simulink model "Md58StEnCtrl"  (R2018b)
settings: Solver=FixedStepDiscrete  StartTime=0.0  StopTime=10.0  FixedStep=0.01  RelTol=1e-3
undefined symbols (not defined in the file or in its folder): data, KeSMSuFirstRwStBackPosDelta_Val, KeSMSuFirstRwStCushFoldPosDelta_Val, KeSMSuFirstRwStFwdBkwdPosDelta_Val, KeSMSw4SSecRwLtStLgrstOtwdInwdClosePos1_Val, KeSMSw4SSecRwLtStLgrstUpwdDnwdClosePos1_Val, KeSMSw4SSecRwLtStLgrstUpwdDnwdClosePos2_Val, KeSMSw4SSecRwLtStLgrstUpwdDnwdOpenPos1_Val, PassStBkReclnEn_Clear, PassStBkReclnEn_Set, PassStCshnFldEn_Clear, PassStCshnFldEn_Set, PassStFwdBkwdEn_Clear, PassStFwdBkwdEn_Set, SecRwRtStBkReclnEn_Clear, SecRwRtStBkReclnEn_Set, SecRwRtStFwdBkwdEn_Clear, SecRwRtStFwdBkwdEn_Set, SecRwRtStLgrstInwdOtwdEn_Clear, SecRwRtStLgrstInwdOtwdEn_Set, SecRwRtStLgrstUpwdDnwdEn_Clear, SecRwRtStLgrstUpwdDnwdEn_Set, ThdRwLtStBkReclnEn_Clear, ThdRwLtStBkReclnEn_Set, ThdRwLtStFwdBkwdEn_Clear, ThdRwLtStFwdBkwdEn_Set, ThdRwRtStBkReclnEn_Clear, ThdRwRtStBkReclnEn_Set, ThdRwRtStFwdBkwdEn_Clear, ThdRwRtStFwdBkwdEn_Set, ZeroREn_Clear, ZeroREn_Set
libraries: simulink x1
(part 1 of 2)
settings Model: Creator=sn2xws  LastModifiedBy=sn2xws
settings Model: ModifiedHistory=|
  | 2024.10.21 V3.0.0 新增Md58
  | 2024.11.18 V3.0.1 CR946473
  | 2024.112.4  V3.0.2 单元测试发现的副驾到位置判断问题
settings DataIOCC: SaveFormat=StructureWithTime
settings OptimizationCC: DefaultParameterBehavior=Inlined  EnhancedBackFolding=on  PassReuseOutputArgsAs=Individual arguments  ZeroExternalMemoryAtStartup=off  ZeroInternalMemoryAtStartup=off  OptimizeBlockOrder=speed  DifferentSizesBufferReuse=on  OptimizationCustomize=off
settings DebuggingCC: ParameterTunabilityLossMsg=error
settings SFSimCC: MATLABDynamicMemAlloc=off
settings RTWCC: SystemTargetFile=autosar.tlc  GenCodeOnly=on  TemplateMakefile=ert_default_tmf  Description=AUTOSAR  GenerateReport=on  IncludeHyperlinkInReport=on  LaunchReport=on  GenerateTraceInfo=on  GenerateTraceReport=on  GenerateTraceReportSl=on  GenerateTraceReportSf=on  GenerateTraceReportEml=on
settings CodeAppCC: ForceParamTrailComments=on  IgnoreCustomStorageClasses=off  OperatorAnnotations=on  SimulinkDataObjDesc=on  SFDataObjDesc=on  InsertBlockDesc=on
settings STFCustomTargetCC: TargetLangStandard=C99 (ISO)  MultiwordLength=256  ParMdlRefBuildCompliant=on  CompOptLevelCompliant=on  IncludeMdlTerminateFcn=off  CombineOutputUpdateFcns=on  SuppressErrorStatus=on  ERTCustomFileBanners=on  SupportNonFinite=off  SupportComplex=off  SupportContinuousTime=off  SupportNonInlinedSFcns=off  RemoveResetFunc=on  MATLABClassNameForMDSCustomization=Simulink.SoftwareTarget.ERTCustomization  AutosarCompliant=on  UseToolchainInfoCompliant=on  LookupTableObjectStructAxisOrder=2,1,3,4,...  LUTObjectStructOrderEvenSpacing=Size,Table,Breakpoints  SystemTargetFile=autosar.tlc
settings ERTTargetCC: TargetLangStandard=C99 (ISO)  ConcurrentExecutionCompliant=off  IncludeMdlTerminateFcn=off  SuppressErrorStatus=on  SupportNonFinite=off  SupportComplex=off  ModelStepFunctionPrototypeControlCompliant=off  CPPClassGenCompliant=off  AutosarCompliant=on  LookupTableObjectStructAxisOrder=2,1,3,4,...  LUTObjectStructOrderEvenSpacing=Size,Table,Breakpoints  InlinedParameterPlacement=NonHierarchical  ERTCustomFileTemplate=example_file_process.tlc  ERTFilePackagingFormat=Compact

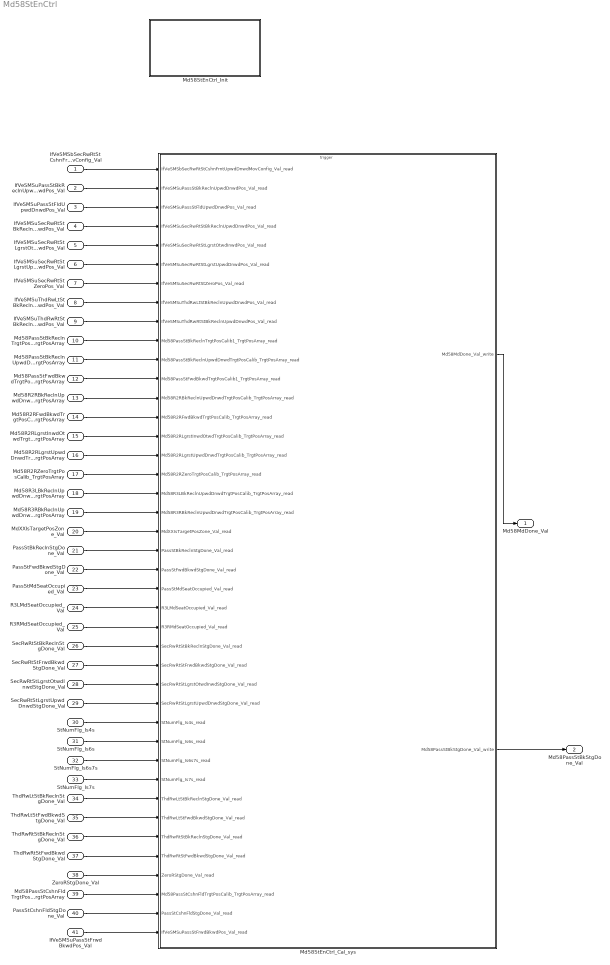
== system Md58StEnCtrl ==
  IfVeSMSbSecRwRtStCshnFrntUpwdDnwdMovConfig_Val : Inport  OutDataTypeStr=boolean  PortDimensions=1
  IfVeSMSuPassStBkReclnUpwdDnwdPos_Val : Inport  Port=2  OutDataTypeStr=uint16  PortDimensions=1
  IfVeSMSuPassStFldUpwdDnwdPos_Val : Inport  Port=3  OutDataTypeStr=uint16  PortDimensions=1
  IfVeSMSuSecRwRtStBkReclnUpwdDnwdPos_Val : Inport  Port=4  OutDataTypeStr=uint16  PortDimensions=1
  IfVeSMSuSecRwRtStLgrstOtwdInwdPos_Val : Inport  Port=5  OutDataTypeStr=uint16  PortDimensions=1
  IfVeSMSuSecRwRtStLgrstUpwdDnwdPos_Val : Inport  Port=6  OutDataTypeStr=uint16  PortDimensions=1
  IfVeSMSuSecRwRtStZeroPos_Val : Inport  Port=7  OutDataTypeStr=uint16  PortDimensions=1
  IfVeSMSuThdRwLtStBkReclnUpwdDnwdPos_Val : Inport  Port=8  OutDataTypeStr=uint16  PortDimensions=1
  IfVeSMSuThdRwRtStBkReclnUpwdDnwdPos_Val : Inport  Port=9  OutDataTypeStr=uint16  PortDimensions=1
  Md58PassStBkReclnTrgtPosCalib1_TrgtPosArray : Inport  Description=|  Port=10  OutDataTypeStr=uint16  PortDimensions=3
      | 0:Pos
      | 1:Max
      | 2:Min
  Md58PassStBkReclnUpwdDnwdTrgtPosCalib_TrgtPosArray : Inport  Description=|  Port=11  OutDataTypeStr=uint16  PortDimensions=3
      | 0:Pos
      | 1:Max
      | 2:Min
  Md58PassStFwdBkwdTrgtPosCalib1_TrgtPosArray : Inport  Description=|  Port=12  OutDataTypeStr=uint16  PortDimensions=3
      | 0:Pos
      | 1:Max
      | 2:Min
  Md58R2RBkReclnUpwdDnwdTrgtPosCalib_TrgtPosArray : Inport  Description=|  Port=13  OutDataTypeStr=uint16  PortDimensions=3
      | 0:Pos
      | 1:Max
      | 2:Min
  Md58R2RFwdBkwdTrgtPosCalib_TrgtPosArray : Inport  Description=|  Port=14  OutDataTypeStr=uint16  PortDimensions=3
      | 0:Pos
      | 1:Max
      | 2:Min
  Md58R2RLgrstInwdOtwdTrgtPosCalib_TrgtPosArray : Inport  Description=|  Port=15  OutDataTypeStr=uint16  PortDimensions=3
      | 0:Pos
      | 1:Max
      | 2:Min
  Md58R2RLgrstUpwdDnwdTrgtPosCalib_TrgtPosArray : Inport  Description=|  Port=16  OutDataTypeStr=uint16  PortDimensions=3
      | 0:Pos
      | 1:Max
      | 2:Min
  Md58R2RZeroTrgtPosCalib_TrgtPosArray : Inport  Description=|  Port=17  OutDataTypeStr=uint16  PortDimensions=3
      | 0:Pos
      | 1:Max
      | 2:Min
  Md58R3LBkReclnUpwdDnwdTrgtPosCalib_TrgtPosArray : Inport  Description=|  Port=18  OutDataTypeStr=uint16  PortDimensions=3
      | 0:Pos
      | 1:Max
      | 2:Min
  Md58R3RBkReclnUpwdDnwdTrgtPosCalib_TrgtPosArray : Inport  Description=|  Port=19  OutDataTypeStr=uint16  PortDimensions=3
      | 0:Pos
      | 1:Max
      | 2:Min
  MdXXIsTargetPosZone_Val : Inport  Port=20  OutDataTypeStr=uint32  PortDimensions=1
  PassStBkReclnStgDone_Val : Inport  Port=21  OutDataTypeStr=boolean  PortDimensions=1
  PassStFwdBkwdStgDone_Val : Inport  Port=22  OutDataTypeStr=boolean  PortDimensions=1
  PassStMdSeatOccupied_Val : Inport  Port=23  OutDataTypeStr=boolean  PortDimensions=1
  R3LMdSeatOccupied_Val : Inport  Port=24  OutDataTypeStr=boolean  PortDimensions=1
  R3RMdSeatOccupied_Val : Inport  Port=25  OutDataTypeStr=boolean  PortDimensions=1
  SecRwRtStBkReclnStgDone_Val : Inport  Port=26  OutDataTypeStr=boolean  PortDimensions=1
  SecRwRtStFrwdBkwdStgDone_Val : Inport  Port=27  OutDataTypeStr=boolean  PortDimensions=1
  SecRwRtStLgrstOtwdInwdStgDone_Val : Inport  Port=28  OutDataTypeStr=boolean  PortDimensions=1
  SecRwRtStLgrstUpwdDnwdStgDone_Val : Inport  Port=29  OutDataTypeStr=boolean  PortDimensions=1
  StNumFlg_Is4s : Inport  Port=30  OutDataTypeStr=boolean  PortDimensions=1
  StNumFlg_Is6s : Inport  Port=31  OutDataTypeStr=boolean  PortDimensions=1
  StNumFlg_Is6s7s : Inport  Port=32  OutDataTypeStr=boolean  PortDimensions=1
  StNumFlg_Is7s : Inport  Port=33  OutDataTypeStr=boolean  PortDimensions=1
  ThdRwLtStBkReclnStgDone_Val : Inport  Port=34  OutDataTypeStr=boolean  PortDimensions=1
  ThdRwLtStFwdBkwdStgDone_Val : Inport  Port=35  OutDataTypeStr=boolean  PortDimensions=1
  ThdRwRtStBkReclnStgDone_Val : Inport  Port=36  OutDataTypeStr=boolean  PortDimensions=1
  ThdRwRtStFwdBkwdStgDone_Val : Inport  Port=37  OutDataTypeStr=boolean  PortDimensions=1
  ZeroRStgDone_Val : Inport  Port=38  OutDataTypeStr=boolean  PortDimensions=1
  Md58PassStCshnFldTrgtPosCalib_TrgtPosArray : Inport  Description=|  Port=39  OutDataTypeStr=uint16  PortDimensions=3
      | 0:Pos
      | 1:Max
      | 2:Min
  PassStCshnFldStgDone_Val : Inport  Port=40  OutDataTypeStr=boolean  PortDimensions=1
  IfVeSMSuPassStFrwdBkwdPos_Val : Inport  Port=41  OutDataTypeStr=uint16  PortDimensions=1
  Md58StEnCtrl_Cal_sys : Subsystem
  Md58StEnCtrl_Init : Subsystem
  Md58MdDone_Val : Outport  OutDataTypeStr=uint8  PortDimensions=1
  Md58PassStBkStgDone_Val : Outport  Port=2  OutDataTypeStr=boolean  PortDimensions=1
  wires:
  IfVeSMSbSecRwRtStCshnFrntUpwdDnwdMovConfig_Val/1 -> Md58StEnCtrl_Cal_sys/1(IfVeSMSbSecRwRtStCshnFrntUpwdDnwdMovConfig_Val_read)
  IfVeSMSuPassStBkReclnUpwdDnwdPos_Val/1 -> Md58StEnCtrl_Cal_sys/2(IfVeSMSuPassStBkReclnUpwdDnwdPos_Val_read)
  IfVeSMSuPassStFldUpwdDnwdPos_Val/1 -> Md58StEnCtrl_Cal_sys/3(IfVeSMSuPassStFldUpwdDnwdPos_Val_read)
  IfVeSMSuSecRwRtStBkReclnUpwdDnwdPos_Val/1 -> Md58StEnCtrl_Cal_sys/4(IfVeSMSuSecRwRtStBkReclnUpwdDnwdPos_Val_read)
  IfVeSMSuSecRwRtStLgrstOtwdInwdPos_Val/1 -> Md58StEnCtrl_Cal_sys/5(IfVeSMSuSecRwRtStLgrstOtwdInwdPos_Val_read)
  IfVeSMSuSecRwRtStLgrstUpwdDnwdPos_Val/1 -> Md58StEnCtrl_Cal_sys/6(IfVeSMSuSecRwRtStLgrstUpwdDnwdPos_Val_read)
  IfVeSMSuSecRwRtStZeroPos_Val/1 -> Md58StEnCtrl_Cal_sys/7(IfVeSMSuSecRwRtStZeroPos_Val_read)
  IfVeSMSuThdRwLtStBkReclnUpwdDnwdPos_Val/1 -> Md58StEnCtrl_Cal_sys/8(IfVeSMSuThdRwLtStBkReclnUpwdDnwdPos_Val_read)
  IfVeSMSuThdRwRtStBkReclnUpwdDnwdPos_Val/1 -> Md58StEnCtrl_Cal_sys/9(IfVeSMSuThdRwRtStBkReclnUpwdDnwdPos_Val_read)
  Md58PassStBkReclnTrgtPosCalib1_TrgtPosArray/1 -> Md58StEnCtrl_Cal_sys/10(Md58PassStBkReclnTrgtPosCalib1_TrgtPosArray_read)
  Md58PassStBkReclnUpwdDnwdTrgtPosCalib_TrgtPosArray/1 -> Md58StEnCtrl_Cal_sys/11(Md58PassStBkReclnUpwdDnwdTrgtPosCalib_TrgtPosArray_read)
  Md58PassStFwdBkwdTrgtPosCalib1_TrgtPosArray/1 -> Md58StEnCtrl_Cal_sys/12(Md58PassStFwdBkwdTrgtPosCalib1_TrgtPosArray_read)
  Md58R2RBkReclnUpwdDnwdTrgtPosCalib_TrgtPosArray/1 -> Md58StEnCtrl_Cal_sys/13(Md58R2RBkReclnUpwdDnwdTrgtPosCalib_TrgtPosArray_read)
  Md58R2RFwdBkwdTrgtPosCalib_TrgtPosArray/1 -> Md58StEnCtrl_Cal_sys/14(Md58R2RFwdBkwdTrgtPosCalib_TrgtPosArray_read)
  Md58R2RLgrstInwdOtwdTrgtPosCalib_TrgtPosArray/1 -> Md58StEnCtrl_Cal_sys/15(Md58R2RLgrstInwdOtwdTrgtPosCalib_TrgtPosArray_read)
  Md58R2RLgrstUpwdDnwdTrgtPosCalib_TrgtPosArray/1 -> Md58StEnCtrl_Cal_sys/16(Md58R2RLgrstUpwdDnwdTrgtPosCalib_TrgtPosArray_read)
  Md58R2RZeroTrgtPosCalib_TrgtPosArray/1 -> Md58StEnCtrl_Cal_sys/17(Md58R2RZeroTrgtPosCalib_TrgtPosArray_read)
  Md58R3LBkReclnUpwdDnwdTrgtPosCalib_TrgtPosArray/1 -> Md58StEnCtrl_Cal_sys/18(Md58R3LBkReclnUpwdDnwdTrgtPosCalib_TrgtPosArray_read)
  Md58R3RBkReclnUpwdDnwdTrgtPosCalib_TrgtPosArray/1 -> Md58StEnCtrl_Cal_sys/19(Md58R3RBkReclnUpwdDnwdTrgtPosCalib_TrgtPosArray_read)
  MdXXIsTargetPosZone_Val/1 -> Md58StEnCtrl_Cal_sys/20(MdXXIsTargetPosZone_Val_read)
  PassStBkReclnStgDone_Val/1 -> Md58StEnCtrl_Cal_sys/21(PassStBkReclnStgDone_Val_read)
  PassStFwdBkwdStgDone_Val/1 -> Md58StEnCtrl_Cal_sys/22(PassStFwdBkwdStgDone_Val_read)
  PassStMdSeatOccupied_Val/1 -> Md58StEnCtrl_Cal_sys/23(PassStMdSeatOccupied_Val_read)
  R3LMdSeatOccupied_Val/1 -> Md58StEnCtrl_Cal_sys/24(R3LMdSeatOccupied_Val_read)
  R3RMdSeatOccupied_Val/1 -> Md58StEnCtrl_Cal_sys/25(R3RMdSeatOccupied_Val_read)
  SecRwRtStBkReclnStgDone_Val/1 -> Md58StEnCtrl_Cal_sys/26(SecRwRtStBkReclnStgDone_Val_read)
  SecRwRtStFrwdBkwdStgDone_Val/1 -> Md58StEnCtrl_Cal_sys/27(SecRwRtStFrwdBkwdStgDone_Val_read)
  SecRwRtStLgrstOtwdInwdStgDone_Val/1 -> Md58StEnCtrl_Cal_sys/28(SecRwRtStLgrstOtwdInwdStgDone_Val_read)
  SecRwRtStLgrstUpwdDnwdStgDone_Val/1 -> Md58StEnCtrl_Cal_sys/29(SecRwRtStLgrstUpwdDnwdStgDone_Val_read)
  StNumFlg_Is4s/1 -> Md58StEnCtrl_Cal_sys/30(StNumFlg_Is4s_read)
  StNumFlg_Is6s/1 -> Md58StEnCtrl_Cal_sys/31(StNumFlg_Is6s_read)
  StNumFlg_Is6s7s/1 -> Md58StEnCtrl_Cal_sys/32(StNumFlg_Is6s7s_read)
  StNumFlg_Is7s/1 -> Md58StEnCtrl_Cal_sys/33(StNumFlg_Is7s_read)
  ThdRwLtStBkReclnStgDone_Val/1 -> Md58StEnCtrl_Cal_sys/34(ThdRwLtStBkReclnStgDone_Val_read)
  ThdRwLtStFwdBkwdStgDone_Val/1 -> Md58StEnCtrl_Cal_sys/35(ThdRwLtStFwdBkwdStgDone_Val_read)
  ThdRwRtStBkReclnStgDone_Val/1 -> Md58StEnCtrl_Cal_sys/36(ThdRwRtStBkReclnStgDone_Val_read)
  ThdRwRtStFwdBkwdStgDone_Val/1 -> Md58StEnCtrl_Cal_sys/37(ThdRwRtStFwdBkwdStgDone_Val_read)
  ZeroRStgDone_Val/1 -> Md58StEnCtrl_Cal_sys/38(ZeroRStgDone_Val_read)
  Md58StEnCtrl_Cal_sys/1(Md58MdDone_Val_write) -> Md58MdDone_Val/1
  Md58PassStCshnFldTrgtPosCalib_TrgtPosArray/1 -> Md58StEnCtrl_Cal_sys/39(Md58PassStCshnFldTrgtPosCalib_TrgtPosArray_read)
  PassStCshnFldStgDone_Val/1 -> Md58StEnCtrl_Cal_sys/40(PassStCshnFldStgDone_Val_read)
  IfVeSMSuPassStFrwdBkwdPos_Val/1 -> Md58StEnCtrl_Cal_sys/41(IfVeSMSuPassStFrwdBkwdPos_Val_read)
  Md58StEnCtrl_Cal_sys/2(Md58PassStBkStgDone_Val_write) -> Md58PassStBkStgDone_Val/1

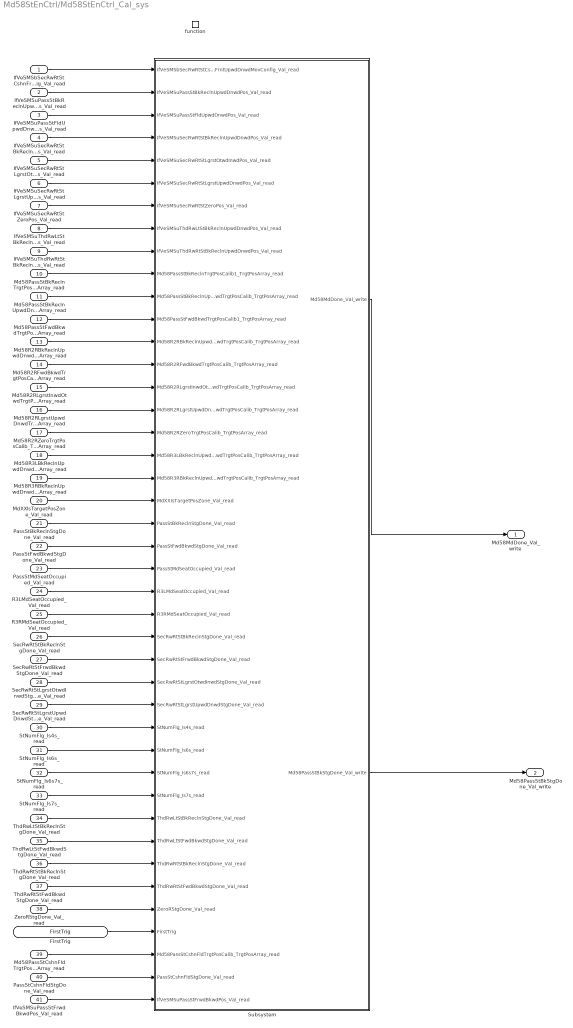
== system Md58StEnCtrl/Md58StEnCtrl_Cal_sys ==
  IfVeSMSbSecRwRtStCshnFrntUpwdDnwdMovConfig_Val_read : Inport
  IfVeSMSuPassStBkReclnUpwdDnwdPos_Val_read : Inport  Port=2
  IfVeSMSuPassStFldUpwdDnwdPos_Val_read : Inport  Port=3
  IfVeSMSuSecRwRtStBkReclnUpwdDnwdPos_Val_read : Inport  Port=4
  IfVeSMSuSecRwRtStLgrstOtwdInwdPos_Val_read : Inport  Port=5
  IfVeSMSuSecRwRtStLgrstUpwdDnwdPos_Val_read : Inport  Port=6
  IfVeSMSuSecRwRtStZeroPos_Val_read : Inport  Port=7
  IfVeSMSuThdRwLtStBkReclnUpwdDnwdPos_Val_read : Inport  Port=8
  IfVeSMSuThdRwRtStBkReclnUpwdDnwdPos_Val_read : Inport  Port=9
  Md58PassStBkReclnTrgtPosCalib1_TrgtPosArray_read : Inport  Port=10
  Md58PassStBkReclnUpwdDnwdTrgtPosCalib_TrgtPosArray_read : Inport  Port=11
  Md58PassStFwdBkwdTrgtPosCalib1_TrgtPosArray_read : Inport  Port=12
  Md58R2RBkReclnUpwdDnwdTrgtPosCalib_TrgtPosArray_read : Inport  Port=13
  Md58R2RFwdBkwdTrgtPosCalib_TrgtPosArray_read : Inport  Port=14
  Md58R2RLgrstInwdOtwdTrgtPosCalib_TrgtPosArray_read : Inport  Port=15
  Md58R2RLgrstUpwdDnwdTrgtPosCalib_TrgtPosArray_read : Inport  Port=16
  Md58R2RZeroTrgtPosCalib_TrgtPosArray_read : Inport  Port=17
  Md58R3LBkReclnUpwdDnwdTrgtPosCalib_TrgtPosArray_read : Inport  Port=18
  Md58R3RBkReclnUpwdDnwdTrgtPosCalib_TrgtPosArray_read : Inport  Port=19
  MdXXIsTargetPosZone_Val_read : Inport  Port=20
  PassStBkReclnStgDone_Val_read : Inport  Port=21
  PassStFwdBkwdStgDone_Val_read : Inport  Port=22
  PassStMdSeatOccupied_Val_read : Inport  Port=23
  R3LMdSeatOccupied_Val_read : Inport  Port=24
  R3RMdSeatOccupied_Val_read : Inport  Port=25
  SecRwRtStBkReclnStgDone_Val_read : Inport  Port=26
  SecRwRtStFrwdBkwdStgDone_Val_read : Inport  Port=27
  SecRwRtStLgrstOtwdInwdStgDone_Val_read : Inport  Port=28
  SecRwRtStLgrstUpwdDnwdStgDone_Val_read : Inport  Port=29
  StNumFlg_Is4s_read : Inport  Port=30
  StNumFlg_Is6s_read : Inport  Port=31
  StNumFlg_Is6s7s_read : Inport  Port=32
  StNumFlg_Is7s_read : Inport  Port=33
  ThdRwLtStBkReclnStgDone_Val_read : Inport  Port=34
  ThdRwLtStFwdBkwdStgDone_Val_read : Inport  Port=35
  ThdRwRtStBkReclnStgDone_Val_read : Inport  Port=36
  ThdRwRtStFwdBkwdStgDone_Val_read : Inport  Port=37
  ZeroRStgDone_Val_read : Inport  Port=38
  Md58PassStCshnFldTrgtPosCalib_TrgtPosArray_read : Inport  Port=39
  PassStCshnFldStgDone_Val_read : Inport  Port=40
  IfVeSMSuPassStFrwdBkwdPos_Val_read : Inport  Port=41
  function : TriggerPort  TriggerType=function-call  IsSimulinkFunction=on  FunctionName=Md58StEnCtrl_Cal  VariantControl=(inherit)
  Subsystem : Subsystem
  FirstTrig : ArgIn  OutDataTypeStr=boolean  ArgumentName=FirstTrig
  Md58MdDone_Val_write : Outport
      settings: EnsureOutportIsVirtual=on
  Md58PassStBkStgDone_Val_write : Outport  Port=2
      settings: EnsureOutportIsVirtual=on
  wires:
  IfVeSMSbSecRwRtStCshnFrntUpwdDnwdMovConfig_Val_read/1 -> Subsystem/1(IfVeSMSbSecRwRtStCshnFrntUpwdDnwdMovConfig_Val_read)
  IfVeSMSuPassStBkReclnUpwdDnwdPos_Val_read/1 -> Subsystem/2(IfVeSMSuPassStBkReclnUpwdDnwdPos_Val_read)
  IfVeSMSuPassStFldUpwdDnwdPos_Val_read/1 -> Subsystem/3(IfVeSMSuPassStFldUpwdDnwdPos_Val_read)
  IfVeSMSuSecRwRtStBkReclnUpwdDnwdPos_Val_read/1 -> Subsystem/4(IfVeSMSuSecRwRtStBkReclnUpwdDnwdPos_Val_read)
  IfVeSMSuSecRwRtStLgrstOtwdInwdPos_Val_read/1 -> Subsystem/5(IfVeSMSuSecRwRtStLgrstOtwdInwdPos_Val_read)
  IfVeSMSuSecRwRtStLgrstUpwdDnwdPos_Val_read/1 -> Subsystem/6(IfVeSMSuSecRwRtStLgrstUpwdDnwdPos_Val_read)
  IfVeSMSuSecRwRtStZeroPos_Val_read/1 -> Subsystem/7(IfVeSMSuSecRwRtStZeroPos_Val_read)
  IfVeSMSuThdRwLtStBkReclnUpwdDnwdPos_Val_read/1 -> Subsystem/8(IfVeSMSuThdRwLtStBkReclnUpwdDnwdPos_Val_read)
  IfVeSMSuThdRwRtStBkReclnUpwdDnwdPos_Val_read/1 -> Subsystem/9(IfVeSMSuThdRwRtStBkReclnUpwdDnwdPos_Val_read)
  Md58PassStBkReclnTrgtPosCalib1_TrgtPosArray_read/1 -> Subsystem/10(Md58PassStBkReclnTrgtPosCalib1_TrgtPosArray_read)
  Md58PassStBkReclnUpwdDnwdTrgtPosCalib_TrgtPosArray_read/1 -> Subsystem/11(Md58PassStBkReclnUpwdDnwdTrgtPosCalib_TrgtPosArray_read)
  Md58PassStFwdBkwdTrgtPosCalib1_TrgtPosArray_read/1 -> Subsystem/12(Md58PassStFwdBkwdTrgtPosCalib1_TrgtPosArray_read)
  Md58R2RBkReclnUpwdDnwdTrgtPosCalib_TrgtPosArray_read/1 -> Subsystem/13(Md58R2RBkReclnUpwdDnwdTrgtPosCalib_TrgtPosArray_read)
  Md58R2RFwdBkwdTrgtPosCalib_TrgtPosArray_read/1 -> Subsystem/14(Md58R2RFwdBkwdTrgtPosCalib_TrgtPosArray_read)
  Md58R2RLgrstInwdOtwdTrgtPosCalib_TrgtPosArray_read/1 -> Subsystem/15(Md58R2RLgrstInwdOtwdTrgtPosCalib_TrgtPosArray_read)
  Md58R2RLgrstUpwdDnwdTrgtPosCalib_TrgtPosArray_read/1 -> Subsystem/16(Md58R2RLgrstUpwdDnwdTrgtPosCalib_TrgtPosArray_read)
  Md58R2RZeroTrgtPosCalib_TrgtPosArray_read/1 -> Subsystem/17(Md58R2RZeroTrgtPosCalib_TrgtPosArray_read)
  Md58R3LBkReclnUpwdDnwdTrgtPosCalib_TrgtPosArray_read/1 -> Subsystem/18(Md58R3LBkReclnUpwdDnwdTrgtPosCalib_TrgtPosArray_read)
  Md58R3RBkReclnUpwdDnwdTrgtPosCalib_TrgtPosArray_read/1 -> Subsystem/19(Md58R3RBkReclnUpwdDnwdTrgtPosCalib_TrgtPosArray_read)
  MdXXIsTargetPosZone_Val_read/1 -> Subsystem/20(MdXXIsTargetPosZone_Val_read)
  PassStBkReclnStgDone_Val_read/1 -> Subsystem/21(PassStBkReclnStgDone_Val_read)
  PassStFwdBkwdStgDone_Val_read/1 -> Subsystem/22(PassStFwdBkwdStgDone_Val_read)
  PassStMdSeatOccupied_Val_read/1 -> Subsystem/23(PassStMdSeatOccupied_Val_read)
  R3LMdSeatOccupied_Val_read/1 -> Subsystem/24(R3LMdSeatOccupied_Val_read)
  R3RMdSeatOccupied_Val_read/1 -> Subsystem/25(R3RMdSeatOccupied_Val_read)
  SecRwRtStBkReclnStgDone_Val_read/1 -> Subsystem/26(SecRwRtStBkReclnStgDone_Val_read)
  SecRwRtStFrwdBkwdStgDone_Val_read/1 -> Subsystem/27(SecRwRtStFrwdBkwdStgDone_Val_read)
  SecRwRtStLgrstOtwdInwdStgDone_Val_read/1 -> Subsystem/28(SecRwRtStLgrstOtwdInwdStgDone_Val_read)
  SecRwRtStLgrstUpwdDnwdStgDone_Val_read/1 -> Subsystem/29(SecRwRtStLgrstUpwdDnwdStgDone_Val_read)
  StNumFlg_Is4s_read/1 -> Subsystem/30(StNumFlg_Is4s_read)
  StNumFlg_Is6s_read/1 -> Subsystem/31(StNumFlg_Is6s_read)
  StNumFlg_Is6s7s_read/1 -> Subsystem/32(StNumFlg_Is6s7s_read)
  StNumFlg_Is7s_read/1 -> Subsystem/33(StNumFlg_Is7s_read)
  ThdRwLtStBkReclnStgDone_Val_read/1 -> Subsystem/34(ThdRwLtStBkReclnStgDone_Val_read)
  ThdRwLtStFwdBkwdStgDone_Val_read/1 -> Subsystem/35(ThdRwLtStFwdBkwdStgDone_Val_read)
  ThdRwRtStBkReclnStgDone_Val_read/1 -> Subsystem/36(ThdRwRtStBkReclnStgDone_Val_read)
  ThdRwRtStFwdBkwdStgDone_Val_read/1 -> Subsystem/37(ThdRwRtStFwdBkwdStgDone_Val_read)
  ZeroRStgDone_Val_read/1 -> Subsystem/38(ZeroRStgDone_Val_read)
  Subsystem/1(Md58MdDone_Val_write) -> Md58MdDone_Val_write/1
  FirstTrig/1 -> Subsystem/39(FirstTrig)
  Md58PassStCshnFldTrgtPosCalib_TrgtPosArray_read/1 -> Subsystem/40(Md58PassStCshnFldTrgtPosCalib_TrgtPosArray_read)
  PassStCshnFldStgDone_Val_read/1 -> Subsystem/41(PassStCshnFldStgDone_Val_read)
  IfVeSMSuPassStFrwdBkwdPos_Val_read/1 -> Subsystem/42(IfVeSMSuPassStFrwdBkwdPos_Val_read)
  Subsystem/2(Md58PassStBkStgDone_Val_write) -> Md58PassStBkStgDone_Val_write/1

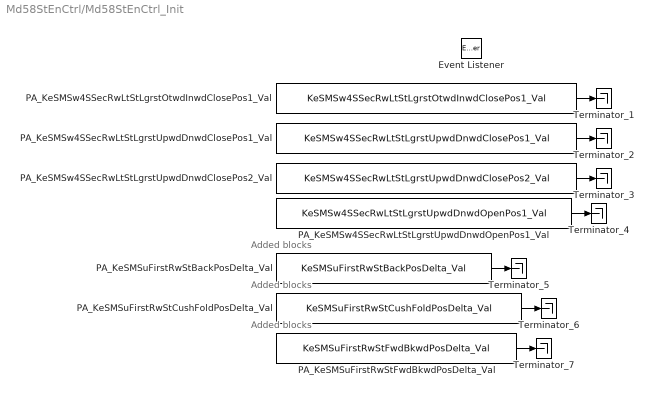
== system Md58StEnCtrl/Md58StEnCtrl_Init ==
  note: Added blocks
  note: Added blocks
  note: Added blocks
  Event Listener : EventListener  EventName=reset
  PA_KeSMSuFirstRwStBackPosDelta_Val : Constant  Value=KeSMSuFirstRwStBackPosDelta_Val
  PA_KeSMSuFirstRwStCushFoldPosDelta_Val : Constant  Value=KeSMSuFirstRwStCushFoldPosDelta_Val
  PA_KeSMSuFirstRwStFwdBkwdPosDelta_Val : Constant  Value=KeSMSuFirstRwStFwdBkwdPosDelta_Val
  PA_KeSMSw4SSecRwLtStLgrstOtwdInwdClosePos1_Val : Constant  Value=KeSMSw4SSecRwLtStLgrstOtwdInwdClosePos1_Val
  PA_KeSMSw4SSecRwLtStLgrstUpwdDnwdClosePos1_Val : Constant  Value=KeSMSw4SSecRwLtStLgrstUpwdDnwdClosePos1_Val
  PA_KeSMSw4SSecRwLtStLgrstUpwdDnwdClosePos2_Val : Constant  Value=KeSMSw4SSecRwLtStLgrstUpwdDnwdClosePos2_Val
  PA_KeSMSw4SSecRwLtStLgrstUpwdDnwdOpenPos1_Val : Constant  Value=KeSMSw4SSecRwLtStLgrstUpwdDnwdOpenPos1_Val
  Terminator_{1..7} (7 alike) : Terminator
  wires:
  PA_KeSMSw4SSecRwLtStLgrstOtwdInwdClosePos1_Val/1 -> Terminator_1/1
  PA_KeSMSw4SSecRwLtStLgrstUpwdDnwdClosePos1_Val/1 -> Terminator_2/1
  PA_KeSMSw4SSecRwLtStLgrstUpwdDnwdClosePos2_Val/1 -> Terminator_3/1
  PA_KeSMSw4SSecRwLtStLgrstUpwdDnwdOpenPos1_Val/1 -> Terminator_4/1
  PA_KeSMSuFirstRwStBackPosDelta_Val/1 -> Terminator_5/1
  PA_KeSMSuFirstRwStCushFoldPosDelta_Val/1 -> Terminator_6/1
  PA_KeSMSuFirstRwStFwdBkwdPosDelta_Val/1 -> Terminator_7/1

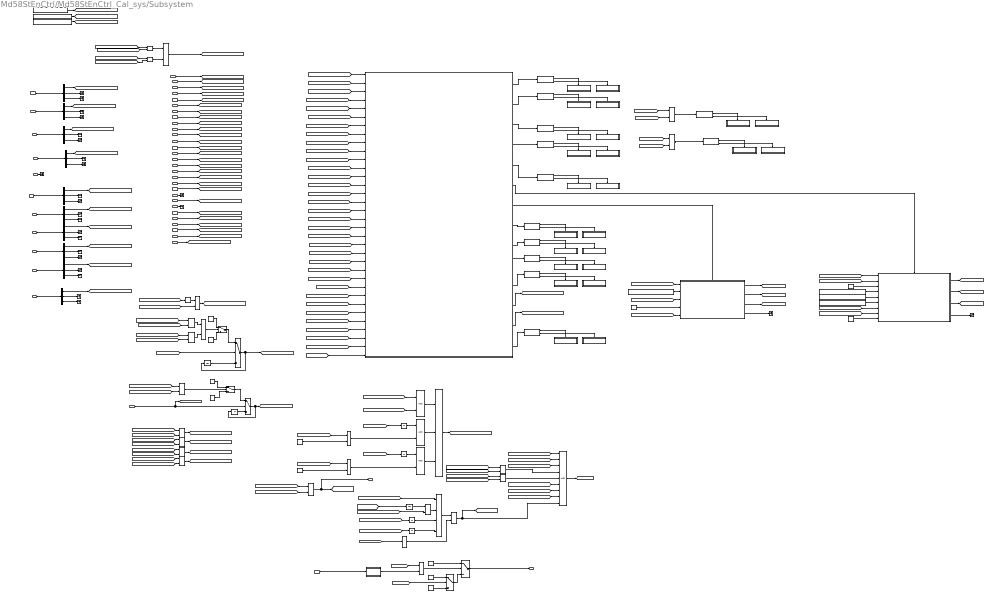
== system Md58StEnCtrl/Md58StEnCtrl_Cal_sys/Subsystem ==
  IfVeSMSbSecRwRtStCshnFrntUpwdDnwdMovConfig_Val_read : Inport
  IfVeSMSuPassStBkReclnUpwdDnwdPos_Val_read : Inport  Port=2
  IfVeSMSuPassStFldUpwdDnwdPos_Val_read : Inport  Port=3
  IfVeSMSuSecRwRtStBkReclnUpwdDnwdPos_Val_read : Inport  Port=4
  IfVeSMSuSecRwRtStLgrstOtwdInwdPos_Val_read : Inport  Port=5
  IfVeSMSuSecRwRtStLgrstUpwdDnwdPos_Val_read : Inport  Port=6
  IfVeSMSuSecRwRtStZeroPos_Val_read : Inport  Port=7
  IfVeSMSuThdRwLtStBkReclnUpwdDnwdPos_Val_read : Inport  Port=8
  IfVeSMSuThdRwRtStBkReclnUpwdDnwdPos_Val_read : Inport  Port=9
  Md58PassStBkReclnTrgtPosCalib1_TrgtPosArray_read : Inport  Port=10
  Md58PassStBkReclnUpwdDnwdTrgtPosCalib_TrgtPosArray_read : Inport  Port=11
  Md58PassStFwdBkwdTrgtPosCalib1_TrgtPosArray_read : Inport  Port=12
  Md58R2RBkReclnUpwdDnwdTrgtPosCalib_TrgtPosArray_read : Inport  Port=13
  Md58R2RFwdBkwdTrgtPosCalib_TrgtPosArray_read : Inport  Port=14
  Md58R2RLgrstInwdOtwdTrgtPosCalib_TrgtPosArray_read : Inport  Port=15
  Md58R2RLgrstUpwdDnwdTrgtPosCalib_TrgtPosArray_read : Inport  Port=16
  Md58R2RZeroTrgtPosCalib_TrgtPosArray_read : Inport  Port=17
  Md58R3LBkReclnUpwdDnwdTrgtPosCalib_TrgtPosArray_read : Inport  Port=18
  Md58R3RBkReclnUpwdDnwdTrgtPosCalib_TrgtPosArray_read : Inport  Port=19
  MdXXIsTargetPosZone_Val_read : Inport  Port=20
  PassStBkReclnStgDone_Val_read : Inport  Port=21
  PassStFwdBkwdStgDone_Val_read : Inport  Port=22
  PassStMdSeatOccupied_Val_read : Inport  Port=23
  R3LMdSeatOccupied_Val_read : Inport  Port=24
  R3RMdSeatOccupied_Val_read : Inport  Port=25
  SecRwRtStBkReclnStgDone_Val_read : Inport  Port=26
  SecRwRtStFrwdBkwdStgDone_Val_read : Inport  Port=27
  SecRwRtStLgrstOtwdInwdStgDone_Val_read : Inport  Port=28
  SecRwRtStLgrstUpwdDnwdStgDone_Val_read : Inport  Port=29
  StNumFlg_Is4s_read : Inport  Port=30
  StNumFlg_Is6s_read : Inport  Port=31
  StNumFlg_Is6s7s_read : Inport  Port=32
  StNumFlg_Is7s_read : Inport  Port=33
  ThdRwLtStBkReclnStgDone_Val_read : Inport  Port=34
  ThdRwLtStFwdBkwdStgDone_Val_read : Inport  Port=35
  ThdRwRtStBkReclnStgDone_Val_read : Inport  Port=36
  ThdRwRtStFwdBkwdStgDone_Val_read : Inport  Port=37
  ZeroRStgDone_Val_read : Inport  Port=38
  FirstTrig : Inport  Port=39
  Md58PassStCshnFldTrgtPosCalib_TrgtPosArray_read : Inport  Port=40
  PassStCshnFldStgDone_Val_read : Inport  Port=41
  IfVeSMSuPassStFrwdBkwdPos_Val_read : Inport  Port=42
  32BitSelector : Subsystem  mask(32 Bit Selector){BitNum=21}
      mask prompts: BitNum "Select Bit Number"
      mask help: Allows selection of a particular bit (0-31) out of a packed word up to 32 bits long. Output will be true if the bit number selected via the mask parameter is equal to one.
      mask TypeOptions BitNum: 0 | 1 | 2 | 3 | 4 | 5 | 6 | 7 | 8 | 9 | 10 | 11 | 12 | 13 | 14 | 15 | 16 | 17 | 18 | 19 | 20 | 21 | 22 | 23 | 24 | 25 | 26 | 27 | 28 | 29 | 30 | 31
      mask Display:
      | text(0.5, 0.8,'BIT','horizontalAlignment','center')
      | text(0.5, 0.5,'SELECTOR','horizontalAlignment','center')
      | text(0.5, 0.2,['-- Bit ',char(get_param(gcb,'BitNum')),' --'],'horizontalAlignment','center')
  Chart : Stateflow chart  TreatAsAtomicUnit=on
  Constant : Constant  OutDataTypeStr=uint8
  Constant1 : Constant  Value=2  OutDataTypeStr=uint8
  Constant10 : Constant  OutDataTypeStr=uint8
  Constant11 : Constant  Value=0  OutDataTypeStr=boolean
  Constant2 : Constant  Value=0  OutDataTypeStr=uint8
  Constant3 : Constant  OutDataTypeStr=boolean
  Constant4 : Constant  OutDataTypeStr=boolean
  Constant5 : Constant  Value=0  OutDataTypeStr=uint16
  Constant6 : Constant  OutDataTypeStr=boolean
  Constant7 : Constant  OutDataTypeStr=uint8
  Constant8 : Constant  Value=2  OutDataTypeStr=uint8
  Constant9 : Constant  Value=2  OutDataTypeStr=uint8
  Demux{,1..9} (10 alike) : Demux  Outputs=3
  If Action Subsystem1 : Subsystem  TreatAsAtomicUnit=on
  If Action Subsystem10 : Subsystem  TreatAsAtomicUnit=on
  If Action Subsystem11 : Subsystem  TreatAsAtomicUnit=on
  If Action Subsystem12 : Subsystem  TreatAsAtomicUnit=on
  If Action Subsystem13 : Subsystem  TreatAsAtomicUnit=on
  If Action Subsystem14 : Subsystem  TreatAsAtomicUnit=on
  If Action Subsystem15 : Subsystem  TreatAsAtomicUnit=on
  If Action Subsystem16 : Subsystem  TreatAsAtomicUnit=on
  If Action Subsystem17 : Subsystem  TreatAsAtomicUnit=on
  If Action Subsystem18 : Subsystem  TreatAsAtomicUnit=on
  If Action Subsystem19 : Subsystem  TreatAsAtomicUnit=on
  If Action Subsystem2 : Subsystem  TreatAsAtomicUnit=on
  If Action Subsystem20 : Subsystem  TreatAsAtomicUnit=on
  If Action Subsystem21 : Subsystem  TreatAsAtomicUnit=on
  If Action Subsystem22 : Subsystem  TreatAsAtomicUnit=on
  If Action Subsystem23 : Subsystem  TreatAsAtomicUnit=on
  If Action Subsystem24 : Subsystem  TreatAsAtomicUnit=on
  If Action Subsystem3 : Subsystem  TreatAsAtomicUnit=on
  If Action Subsystem4 : Subsystem  TreatAsAtomicUnit=on
  If Action Subsystem5 : Subsystem  TreatAsAtomicUnit=on
  If Action Subsystem6 : Subsystem  TreatAsAtomicUnit=on
  If Action Subsystem7 : Subsystem  TreatAsAtomicUnit=on
  If Action Subsystem8 : Subsystem  TreatAsAtomicUnit=on
  If Action Subsystem9 : Subsystem  TreatAsAtomicUnit=on
  If{1..12} (12 alike) : If  IfExpression=u1
  LgrstClose : Subsystem
  LgrstOpen : Subsystem
  Logical Operator : Logic  Operator=NOT  AllPortsSameDT=off  OutDataTypeStr=boolean
  Logical Operator{1,3..4,12,15..19} (9 alike) : Logic  Operator=OR  AllPortsSameDT=off  OutDataTypeStr=boolean
  Logical Operator10 : Logic  Inputs=9  AllPortsSameDT=off  OutDataTypeStr=boolean
  Logical Operator{2,6..9,11,14,20,22} (9 alike) : Logic  AllPortsSameDT=off  OutDataTypeStr=boolean
  Logical Operator13 : Logic  Operator=OR  Inputs=4  AllPortsSameDT=off  OutDataTypeStr=boolean
  Logical Operator21 : Logic  Operator=NOT  Inputs=1  AllPortsSameDT=off  OutDataTypeStr=boolean
  Logical Operator5 : Logic  Operator=OR  Inputs=3  AllPortsSameDT=off  OutDataTypeStr=boolean
  PA_KeSMSuFirstRwStBackPosDelta_Val : Constant  Value=KeSMSuFirstRwStBackPosDelta_Val
  PA_KeSMSuFirstRwStCushFoldPosDelta_Val : Constant  Value=KeSMSuFirstRwStCushFoldPosDelta_Val
  PA_KeSMSuFirstRwStFwdBkwdPosDelta_Val : Constant  Value=KeSMSuFirstRwStFwdBkwdPosDelta_Val
  PA_KeSMSw4SSecRwLtStLgrstOtwdInwdClosePos1_Val1 : Constant  Value=KeSMSw4SSecRwLtStLgrstOtwdInwdClosePos1_Val
  PA_KeSMSw4SSecRwLtStLgrstUpwdDnwdClosePos1_Val1 : Constant  Value=KeSMSw4SSecRwLtStLgrstUpwdDnwdClosePos1_Val
  PA_KeSMSw4SSecRwLtStLgrstUpwdDnwdClosePos2_Val1 : Constant  Value=KeSMSw4SSecRwLtStLgrstUpwdDnwdClosePos2_Val
  PA_KeSMSw4SSecRwLtStLgrstUpwdDnwdOpenPos1_Val1 : Constant  Value=KeSMSw4SSecRwLtStLgrstUpwdDnwdOpenPos1_Val
  Relational Operator : RelationalOperator  OutDataTypeStr=boolean  RndMeth=Simplest
  Relational Operator1 : RelationalOperator  Operator===  OutDataTypeStr=boolean  RndMeth=Simplest
  Relational Operator{2,4..6} (4 alike) : RelationalOperator  Operator=<=  OutDataTypeStr=boolean  RndMeth=Simplest
  Relational Operator3 : RelationalOperator  Operator===  OutDataTypeStr=boolean  RndMeth=Simplest
  Switch{,1..5} (6 alike) : Switch  Criteria=u2 > Threshold
  Terminator{,1..21} (22 alike) : Terminator
  Terminator_23 : Terminator
  Terminator_30 : Terminator
  Terminator_32 : Terminator
  Unit Delay{,1..6} (7 alike) : UnitDelay  SampleTime=-1
  Md58MdDone_Val_write : Outport
      settings: EnsureOutportIsVirtual=on
  Md58PassStBkStgDone_Val_write : Outport  Port=2
      settings: EnsureOutportIsVirtual=on
  wires:
  ThdRwLtStBkReclnStgDone_Val_read/1 -> [ThdRwLtStBkReclnStgDone]
  IfVeSMSuThdRwRtStBkReclnUpwdDnwdPos_Val_read/1 -> [IfVeSMSuThdRwRtStBkReclnUpwdDnwdPos]
  IfVeSMSuPassStFldUpwdDnwdPos_Val_read/1 -> [IfVeSMSuPassStFldUpwdDnwdPos]
  IfVeSMSuSecRwRtStBkReclnUpwdDnwdPos_Val_read/1 -> [IfVeSMSuSecRwRtStBkReclnUpwdDnwdPos]
  IfVeSMSuSecRwRtStLgrstUpwdDnwdPos_Val_read/1 -> [IfVeSMSuSecRwRtStLgrstUpwdDnwdPos]
  SecRwRtStLgrstUpwdDnwdStgDone_Val_read/1 -> [SecRwRtStLgrstUpwdDnwdStgDone]
  IfVeSMSuSecRwRtStLgrstOtwdInwdPos_Val_read/1 -> [IfVeSMSuSecRwRtStLgrstOtwdInwdPos]
  StNumFlg_Is4s_read/1 -> Terminator_30/1
  SecRwRtStBkReclnStgDone_Val_read/1 -> [SecRwRtStBkReclnStgDone]
  IfVeSMSuThdRwLtStBkReclnUpwdDnwdPos_Val_read/1 -> [IfVeSMSuThdRwLtStBkReclnUpwdDnwdPos]
  ThdRwLtStFwdBkwdStgDone_Val_read/1 -> [ThdRwLtStFwdBkwdStgDone]
  StNumFlg_Is6s_read/1 -> [is6s]
  R3RMdSeatOccupied_Val_read/1 -> [R3RMdSeatOccupied]
  SecRwRtStLgrstOtwdInwdStgDone_Val_read/1 -> [SecRwRtStLgrstOtwdInwdStgDone]
  StNumFlg_Is7s_read/1 -> [StNumFlg_Is7s]
  Md58PassStBkReclnUpwdDnwdTrgtPosCalib_TrgtPosArray_read/1 -> Demux/1
  PassStBkReclnStgDone_Val_read/1 -> [PassStBkReclnStgDone]
  R3LMdSeatOccupied_Val_read/1 -> [R3LMdSeatOccupied]
  ThdRwRtStFwdBkwdStgDone_Val_read/1 -> [ThdRwRtStFwdBkwdStgDone]
  IfVeSMSuPassStBkReclnUpwdDnwdPos_Val_read/1 -> [IfVeSMSuPassStBkReclnUpwdDnwdPos]
  ZeroRStgDone_Val_read/1 -> [ZeroRStgDone]
  StNumFlg_Is6s7s_read/1 -> Terminator_32/1
  SecRwRtStFrwdBkwdStgDone_Val_read/1 -> [SecRwRtStFrwdBkwdStgDone]
  PassStFwdBkwdStgDone_Val_read/1 -> [PassStFwdBkwdStgDone]
  IfVeSMSbSecRwRtStCshnFrntUpwdDnwdMovConfig_Val_read/1 -> [IfVeSMSbSecRwRtStCshnFrntUpwdDnwdMovConfig]
  32BitSelector/1(y) -> Logical Operator9/2
  [AllDone] -> Logical Operator9/1
  Logical Operator9/1 -> Switch/2
  Switch1/1 -> Switch/3
  Constant/1 -> Switch/1
  MdXXIsTargetPosZone_Val_read/1 -> 32BitSelector/1(x)
  Switch/1 -> Md58MdDone_Val_write/1
  Constant1/1 -> Switch1/1
  [AllDone] -> Switch1/2
  Constant2/1 -> Switch1/3
  Relational Operator3/1 -> Logical Operator7/2
  [is6s] -> Logical Operator15/2
  [ThdRwLtStFwdBkwdStgDoneModify] -> Logical Operator15/1
  Logical Operator15/1 -> Logical Operator10/5
  Logical Operator2/1 -> Logical Operator5/1
  Constant10/1 -> Relational Operator3/2
  [PassStFwdBkwdStgDone] -> Logical Operator11/2
  Constant9/1 -> Relational Operator1/2
  [SecRwRtStBkReclnStgDone] -> Logical Operator10/2
  [LgrstMoveDirection] -> Relational Operator1/1
  [LgrstMoveDirection] -> Relational Operator3/1
  [ZeroRStgDoneModify] -> Logical Operator10/6
  [is6s] -> Logical Operator12/2
  Logical Operator11/1 -> Logical Operator13/2
  [SecRwRtStFrwdBkwdStgDone] -> Logical Operator10/3
  [LgrstStgDone] -> Logical Operator10/1
  [ThdRwRtStFwdBkwdStgDoneModify] -> Logical Operator10/8
  Unit Delay3/1 -> Logical Operator6/1
  [NotMovPassStFlg] -> Logical Operator13/1
  Logical Operator7/1 -> Logical Operator5/3
  Unit Delay4/1 -> Logical Operator7/1
  Logical Operator6/1 -> Logical Operator5/2
  [FailflgCls] -> Unit Delay4/1
  [ThdRwRtStBkReclnStgDoneModify] -> Logical Operator10/7
  [FailflgOpn] -> Unit Delay3/1
  Logical Operator10/1 -> [AllDone]
  Relational Operator1/1 -> Logical Operator6/2
  Logical Operator5/1 -> [LgrstStgDone]
  [ThdRwLtStBkReclnStgDoneModify] -> Logical Operator12/1
  [SecRwRtStLgrstUpwdDnwdStgDone] -> Logical Operator2/1
  Logical Operator12/1 -> Logical Operator10/4
  [SecRwRtStLgrstOtwdInwdStgDone] -> Logical Operator2/2
  Logical Operator18/1 -> [ThdRwRtStBkReclnStgDoneModify]
  Logical Operator16/1 -> [ThdRwLtStBkReclnStgDoneModify]
  Logical Operator19/1 -> [ThdRwRtStFwdBkwdStgDoneModify]
  Logical Operator17/1 -> [ThdRwLtStFwdBkwdStgDoneModify]
  [R3LMdSeatOccupied] -> Logical Operator16/1
  [R3RMdSeatOccupied] -> Logical Operator19/1
  [R3RMdSeatOccupied] -> Logical Operator18/1
  [ThdRwRtStFwdBkwdStgDone] -> Logical Operator19/2
  [ThdRwLtStFwdBkwdStgDone] -> Logical Operator17/2
  [ThdRwRtStBkReclnStgDone] -> Logical Operator18/2
  [ThdRwLtStBkReclnStgDone] -> Logical Operator16/2
  [R3LMdSeatOccupied] -> Logical Operator17/1
  [IfVeSMSuSecRwRtStLgrstUpwdDnwdPos] -> Relational Operator/1
  [VIPRR2RLgrstUpwdDnwdTrgtPos] -> Relational Operator/2
  Switch3/1 -> Unit Delay/1, [LgrstMoveDirection]
  Constant7/1 -> Switch2/1
  Unit Delay/1 -> Switch3/3
  Switch2/1 -> Switch3/1
  Constant8/1 -> Switch2/3
  Relational Operator/1 -> Switch2/2
  IfVeSMSuSecRwRtStZeroPos_Val_read/1 -> [IfVeSMSuSecRwRtStZeroPos]
  Demux/1 -> [VIPRExitPassStBkReclnUpwdDnwdTrgtPos]
  Demux/2 -> Terminator/1
  Demux/3 -> Terminator1/1
  PassStMdSeatOccupied_Val_read/1 -> [NotMovPassStFlg]
  ThdRwRtStBkReclnStgDone_Val_read/1 -> [ThdRwRtStBkReclnStgDone]
  Demux1/3 -> Terminator3/1
  Demux1/2 -> Terminator2/1
  Md58R2RZeroTrgtPosCalib_TrgtPosArray_read/1 -> Demux1/1
  Demux1/1 -> [VIPRMdR2RZeroTrgtPos]
  Md58R3LBkReclnUpwdDnwdTrgtPosCalib_TrgtPosArray_read/1 -> Demux2/1
  Demux2/2 -> Terminator4/1
  Demux2/3 -> Terminator5/1
  Demux3/3 -> Terminator7/1
  Demux3/2 -> Terminator6/1
  Md58R3RBkReclnUpwdDnwdTrgtPosCalib_TrgtPosArray_read/1 -> Demux3/1
  Demux2/1 -> [VIPRExitR3LBkReclnUpwdDnwdTrgtPos]
  Demux3/1 -> [VIPRExitR3RBkReclnUpwdDnwdTrgtPos]
  Demux4/1 -> [VIPRR2RLgrstUpwdDnwdTrgtPos]
  Md58R2RLgrstUpwdDnwdTrgtPosCalib_TrgtPosArray_read/1 -> Demux4/1
  Demux4/2 -> Terminator8/1
  Demux4/3 -> Terminator9/1
  Demux5/3 -> Terminator11/1
  Demux5/2 -> Terminator10/1
  Md58R2RLgrstInwdOtwdTrgtPosCalib_TrgtPosArray_read/1 -> Demux5/1
  Demux5/1 -> [VIPRR2RLgrstInwdOtwdTrgtPos]
  Demux6/1 -> [VIPRR2RBkReclnUpwdDnwdTrgtPos]
  Md58R2RBkReclnUpwdDnwdTrgtPosCalib_TrgtPosArray_read/1 -> Demux6/1
  Demux6/2 -> Terminator12/1
  Demux6/3 -> Terminator13/1
  Logical Operator/1 -> Logical Operator1/1
  [ZeroRStgDone] -> Logical Operator1/2
  Logical Operator1/1 -> [ZeroRStgDoneModify]
  [IfVeSMSbSecRwRtStCshnFrntUpwdDnwdMovConfig] -> Logical Operator/1
  [StNumFlg_Is7s] -> Chart/25(Is7s)
  [VIPRR2RLgrstUpwdDnwdTrgtPos] -> Chart/7(VIPLR2LLgrstUpwdDnwdTrgtPos)
  If10/1 -> If Action Subsystem20/Action
  Chart/9(ThdRwRtStFwdBkwdEn) -> If9/1
  [SecRwRtStLgrstUpwdDnwdStgDone] -> LgrstOpen/3(LgrstUpwdStgDone)
  If6/2 -> If Action Subsystem12/Action
  [LgrstMoveDirection] -> Chart/14(LgrstMoveDirection)
  Chart/2(SecRwLtStFrwdBkwdEn) -> If1/1
  LgrstOpen/3(LgrstUpwdDnwdEn) -> [LgrstUpwdEn2]
  If3/1 -> If Action Subsystem6/Action
  [IfVeSMSuThdRwRtStBkReclnUpwdDnwdPos] -> Chart/15(IfVeSMSuThdRwRtStBkReclnUpwdDnwdPos)
  If8/2 -> If Action Subsystem11/Action
  [IfVeSMSuSecRwRtStZeroPos] -> Chart/9(IfVeSMSuSecRwLtStZeroPos)
  If11/2 -> If Action Subsystem21/Action
  [LgrstUpwdEn3] -> Logical Operator3/2
  Chart/1(SecRwLtStBkReclnEn) -> If8/1
  If1/2 -> If Action Subsystem1/Action
  If10/2 -> If Action Subsystem19/Action
  [VIPRExitPassStBkReclnUpwdDnwdTrgtPos] -> Chart/24(VIPRExitPassStBkReclnUpwdDnwdTrgtPos)
  [IfVeSMSuSecRwRtStLgrstUpwdDnwdPos] -> LgrstOpen/1(LgrstUpwdDnwdPos)
  If11/1 -> If Action Subsystem22/Action
  If9/1 -> If Action Subsystem18/Action
  Chart/11(PassStBkReclnEn) -> If11/1
  [ThdRwLtStBkReclnStgDoneModify] -> Chart/4(ThdRwLtStBkReclnStgDone)
  If9/2 -> If Action Subsystem17/Action
  Chart/10(PassStFwdBkwdEn) -> If10/1
  Chart/8(ThdRwRtStBkReclnEn) -> If7/1
  If7/1 -> If Action Subsystem16/Action
  [ThdRwRtStFwdBkwdStgDoneModify] -> Chart/21(ThdRwRtStFwdBkwdStgDone)
  [VIPRExitR3LBkReclnUpwdDnwdTrgtPos] -> Chart/22(VIPRExitR3LBkReclnUpwdDnwdTrgtPos)
  PA_KeSMSw4SSecRwLtStLgrstUpwdDnwdOpenPos1_Val1/1 -> LgrstOpen/2(LgrstUpwdDnwdOpenPos1)
  [PassStBkReclnStgDone] -> Chart/18(PassStBkReclnStgDone)
  [R3LMdSeatOccupied] -> Chart/11(R3LMdSeatOccupied)
  If7/2 -> If Action Subsystem15/Action
  [PassStFwdBkwdStgDone] -> Chart/19(PassStFwdBkwdStgDone)
  [R3RMdSeatOccupied] -> Chart/17(R3RMdSeatOccupied)
  If3/2 -> If Action Subsystem5/Action
  [NotMovPassStFlg] -> Chart/16(NotMovPassStFlg)
  [IfVeSMSuThdRwLtStBkReclnUpwdDnwdPos] -> Chart/13(IfVeSMSuThdRwLtStBkReclnUpwdDnwdPos)
  LgrstClose/1(Failflg) -> [FailflgCls]
  LgrstClose/4(FtrstEn) -> Terminator14/1
  Logical Operator3/1 -> If4/1
  [ThdRwRtStBkReclnStgDoneModify] -> Chart/20(ThdRwRtStBkReclnStgDone)
  [SecRwRtStFrwdBkwdStgDone] -> Chart/3(SecRwLtStFrwdBkwdStgDone)
  Chart/3(ThdRwLtStBkReclnEn) -> If2/1
  LgrstClose/2(LgrstInwdOtwdEn) -> [LgrstInwdOtwdEn3]
  If4/1 -> If Action Subsystem8/Action
  PA_KeSMSw4SSecRwLtStLgrstUpwdDnwdClosePos1_Val1/1 -> LgrstClose/4(LgrstUpwdDnwdClosePos1)
  [SecRwRtStLgrstOtwdInwdStgDone] -> LgrstOpen/5(LgrstInwdStgDone)
  Chart/6(LgrstClsEn) -> LgrstClose/Enable
  [LgrstUpwdEn2] -> Logical Operator3/1
  [IfVeSMSuSecRwRtStBkReclnUpwdDnwdPos] -> Chart/1(IfVeSMSuSecRwLtStBkReclnUpwdDnwdPos)
  If4/2 -> If Action Subsystem7/Action
  If5/2 -> If Action Subsystem9/Action
  If2/1 -> If Action Subsystem4/Action
  [LgrstStgDone] -> Chart/12(LgrstStgDone)
  If1/1 -> If Action Subsystem2/Action
  If6/1 -> If Action Subsystem13/Action
  [LgrstInwdOtwdEn2] -> Logical Operator4/1
  [VIPRExitR3RBkReclnUpwdDnwdTrgtPos] -> Chart/23(VIPRExitR3RBkReclnUpwdDnwdTrgtPos)
  Constant3/1 -> LgrstOpen/4(FtrstStgDone)
  [SecRwRtStLgrstUpwdDnwdStgDone] -> LgrstClose/8(LgrstUpwdStgDone)
  LgrstOpen/1(Failflg) -> [FailflgOpn]
  [LgrstInwdOtwdEn3] -> Logical Operator4/2
  [IfVeSMSuSecRwRtStLgrstUpwdDnwdPos] -> LgrstClose/1(LgrstUpwdDnwdPos)
  [ThdRwLtStFwdBkwdStgDoneModify] -> Chart/5(ThdRwLtStFwdBkwdStgDone)
  If5/1 -> If Action Subsystem10/Action
  If8/1 -> If Action Subsystem14/Action
  [ZeroRStgDoneModify] -> Chart/8(ZeroLStgDone)
  PA_KeSMSw4SSecRwLtStLgrstUpwdDnwdClosePos2_Val1/1 -> LgrstClose/5(LgrstUpwdDnwdClosePos2)
  [VIPRMdR2RZeroTrgtPos] -> Chart/10(VIPLMdR2LZeroTrgtPos)
  LgrstOpen/2(LgrstInwdOtwdEn) -> [LgrstInwdOtwdEn2]
  Logical Operator4/1 -> If5/1
  LgrstOpen/4(FtrstEn) -> Terminator15/1
  Constant5/1 -> LgrstClose/3(FtupwdDnwdPos)
  PA_KeSMSw4SSecRwLtStLgrstOtwdInwdClosePos1_Val1/1 -> LgrstClose/6(LgrstInwdOtWdPos1)
  [SecRwRtStBkReclnStgDone] -> Chart/2(SecRwLtStBkReclnStgDone)
  Chart/4(ThdRwLtStFwdBkwdEn) -> If3/1
  [SecRwRtStLgrstOtwdInwdStgDone] -> LgrstClose/7(LgrstInwdStgDone)
  Chart/7(LgrstOpnEn) -> LgrstOpen/Enable
  Chart/5(ZeroLEn) -> If6/1
  LgrstClose/3(LgrstUpwdDnwdEn) -> [LgrstUpwdEn3]
  If2/2 -> If Action Subsystem3/Action
  [VIPRR2RBkReclnUpwdDnwdTrgtPos] -> Chart/6(VIPLR2LBkReclnUpwdDnwdTrgtPos)
  Constant4/1 -> LgrstClose/9(FtrstStgDone)
  [IfVeSMSuSecRwRtStLgrstOtwdInwdPos] -> LgrstClose/2(LgrstInwdOtwdPos)
  Demux7/3 -> Terminator17/1
  Demux7/2 -> Terminator16/1
  Demux7/1 -> [PassStBkReclnUpwdDnwdTrgtPos1]
  Md58PassStBkReclnTrgtPosCalib1_TrgtPosArray_read/1 -> Demux7/1
  Md58PassStFwdBkwdTrgtPosCalib1_TrgtPosArray_read/1 -> Demux8/1
  Demux8/1 -> [Md58PassStFwdBkwdTrgtPos1]
  Demux8/2 -> Terminator18/1
  Demux8/3 -> Terminator19/1
  [PassStCshnFldTrgtPos] -> Relational Operator2/1
  Relational Operator2/1 -> Logical Operator8/1
  Relational Operator4/1 -> Logical Operator8/2
  [VIPRExitPassStBkReclnUpwdDnwdTrgtPos] -> Relational Operator4/1
  Logical Operator8/1 -> [PassStFldTrgt]
  FirstTrig/1 -> [FirstTrig], Switch3/2
  [FirstTrig] -> Switch4/2
  Switch4/1 -> Unit Delay1/1, [FirstPassFldFlg]
  Unit Delay1/1 -> Switch4/3
  [IfVeSMSuPassStFldUpwdDnwdPos] -> Relational Operator5/1
  [IfVeSMSuPassStBkReclnUpwdDnwdPos] -> Relational Operator6/1
  Relational Operator5/1 -> Logical Operator14/1
  Relational Operator6/1 -> Logical Operator14/2
  Logical Operator14/1 -> Switch5/2
  Switch5/1 -> Switch4/1
  Constant6/1 -> Switch5/1
  Constant11/1 -> Switch5/3
  [FirstPassFldFlg] -> Chart/26(FirstPassFldFlg)
  [PassStFldTrgt] -> Chart/27(PassStFldTrgt)
  [Md58PassStFwdBkwdTrgtPos1] -> Chart/29(PassStFwdBkwdTrgtPos1)
  [PassStBkReclnUpwdDnwdTrgtPos1] -> Chart/28(PassStBkReclnUpwdDnwdTrgtPos1)
  Md58R2RFwdBkwdTrgtPosCalib_TrgtPosArray_read/1 -> Terminator_23/1
  Chart/12(PassStFwdBkwdFailflg) -> [PassStFwdBkwdFailflg]
  Chart/13(PassStCshnFldFailflg) -> [PassStCshnFldFailflg]
  [PassStCushFldPosDelta] -> Relational Operator2/2
  [PassStBackPosDelta] -> Relational Operator4/2
  [PassStCushFldPosDelta] -> Relational Operator5/2
  [PassStBackPosDelta] -> Relational Operator6/2
  Md58PassStCshnFldTrgtPosCalib_TrgtPosArray_read/1 -> Demux9/1
  Demux9/2 -> Terminator20/1
  Demux9/3 -> Terminator21/1
  Demux9/1 -> [PassStCshnFldTrgtPos]
  PA_KeSMSuFirstRwStBackPosDelta_Val/1 -> [PassStBackPosDelta]
  PA_KeSMSuFirstRwStCushFoldPosDelta_Val/1 -> [PassStCushFldPosDelta]
  PA_KeSMSuFirstRwStFwdBkwdPosDelta_Val/1 -> [PassStFwdBkwdPosDelta]
  PassStCshnFldStgDone_Val_read/1 -> [PassStCshnFldStgDone]
  [PassStCshnFldFailflg] -> Unit Delay5/1
  [PassStCshnFldStgDone] -> Chart/32(PassStCshnFldStgDone)
  [PassStFwdBkwdPosDelta] -> Chart/31(KeSMSuFirstRwStFwdBkwdPosDelta)
  Chart/14(PassStCshnFldEn) -> If12/1
  If12/1 -> If Action Subsystem24/Action
  If12/2 -> If Action Subsystem23/Action
  [IfVeSMSuPassStFrwdBkwdPos] -> Chart/30(PassStFwdBkwdPos)
  IfVeSMSuPassStFrwdBkwdPos_Val_read/1 -> [IfVeSMSuPassStFrwdBkwdPos]
  [IfVeSMSuPassStBkReclnUpwdDnwdPos] -> Chart/33(PassStBkReclnUpwdDnwdPos)
  [PassStBkReclnStgDone] -> Logical Operator20/1
  [PassStCshnFldStgDone] -> Logical Operator20/2
  Logical Operator20/1 -> Md58PassStBkStgDone_Val_write/1, [Md58PassStBkStgDone]
  [Md58PassStBkStgDone] -> Unit Delay6/1
  Unit Delay6/1 -> Logical Operator11/1
  [PassStFwdBkwdFailflg] -> Unit Delay2/1
  [FirstTrig] -> Logical Operator21/1
  Logical Operator21/1 -> Logical Operator22/2
  [PassStDone] -> Chart/34(PassStDone)
  Unit Delay2/1 -> Logical Operator13/3
  Unit Delay5/1 -> Logical Operator13/4
  Logical Operator13/1 -> Logical Operator22/1
  Logical Operator22/1 -> [PassStDone], Logical Operator10/9

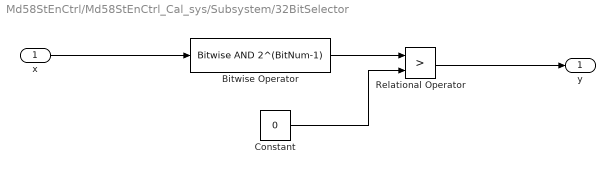
== system Md58StEnCtrl/Md58StEnCtrl_Cal_sys/Subsystem/32BitSelector ==
  x : Inport
  Bitwise Operator : simulink/Logic and Bit Operations/Bitwise Operator  logicop=AND  UseBitMask=on  BitMask=2^(BitNum-1)  BitMaskRealWorld=Stored Integer
  Constant : Constant  Value=0  OutDataTypeStr=uint32
  Relational Operator : RelationalOperator  Operator=>  OutDataTypeStr=boolean  RndMeth=Simplest
  y : Outport
  wires:
  Relational Operator/1 -> y/1
  Constant/1 -> Relational Operator/2
  x/1 -> Bitwise Operator/1
  Bitwise Operator/1 -> Relational Operator/1

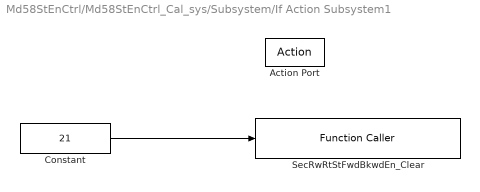
== system Md58StEnCtrl/Md58StEnCtrl_Cal_sys/Subsystem/If Action Subsystem1 ==
  Action Port : ActionPort  ActionType=else
  Constant : Constant  Value=21  OutDataTypeStr=uint8
  SecRwRtStFwdBkwdEn_Clear : FunctionCaller  FunctionPrototype=SecRwRtStFwdBkwdEn_Clear(data)  InputArgumentSpecifications=uint8(1)
  wires:
  Constant/1 -> SecRwRtStFwdBkwdEn_Clear/1

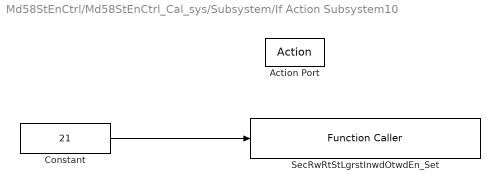
== system Md58StEnCtrl/Md58StEnCtrl_Cal_sys/Subsystem/If Action Subsystem10 ==
  Action Port : ActionPort  ActionType=then
  Constant : Constant  Value=21  OutDataTypeStr=uint8
  SecRwRtStLgrstInwdOtwdEn_Set : FunctionCaller  FunctionPrototype=SecRwRtStLgrstInwdOtwdEn_Set(data)  InputArgumentSpecifications=uint8(1)
  wires:
  Constant/1 -> SecRwRtStLgrstInwdOtwdEn_Set/1

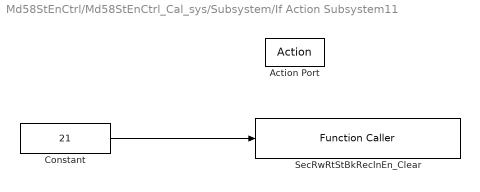
== system Md58StEnCtrl/Md58StEnCtrl_Cal_sys/Subsystem/If Action Subsystem11 ==
  Action Port : ActionPort  ActionType=else
  Constant : Constant  Value=21  OutDataTypeStr=uint8
  SecRwRtStBkReclnEn_Clear : FunctionCaller  FunctionPrototype=SecRwRtStBkReclnEn_Clear(data)  InputArgumentSpecifications=uint8(1)
  wires:
  Constant/1 -> SecRwRtStBkReclnEn_Clear/1

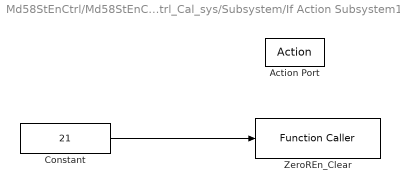
== system Md58StEnCtrl/Md58StEnCtrl_Cal_sys/Subsystem/If Action Subsystem12 ==
  Action Port : ActionPort  ActionType=else
  Constant : Constant  Value=21  OutDataTypeStr=uint8
  ZeroREn_Clear : FunctionCaller  FunctionPrototype=ZeroREn_Clear(data)  InputArgumentSpecifications=uint8(1)
  wires:
  Constant/1 -> ZeroREn_Clear/1

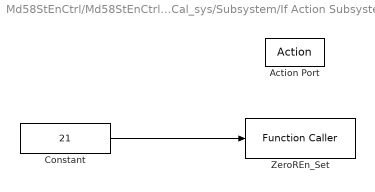
== system Md58StEnCtrl/Md58StEnCtrl_Cal_sys/Subsystem/If Action Subsystem13 ==
  Action Port : ActionPort  ActionType=then
  Constant : Constant  Value=21  OutDataTypeStr=uint8
  ZeroREn_Set : FunctionCaller  FunctionPrototype=ZeroREn_Set(data)  InputArgumentSpecifications=uint8(1)
  wires:
  Constant/1 -> ZeroREn_Set/1

== system Md58StEnCtrl/Md58StEnCtrl_Cal_sys/Subsystem/If Action Subsystem14 ==
  Action Port : ActionPort  ActionType=then
  Constant : Constant  Value=21  OutDataTypeStr=uint8
  SecRwRtStBkReclnEn_Set : FunctionCaller  FunctionPrototype=SecRwRtStBkReclnEn_Set(data)  InputArgumentSpecifications=uint8(1)
  wires:
  Constant/1 -> SecRwRtStBkReclnEn_Set/1

== system Md58StEnCtrl/Md58StEnCtrl_Cal_sys/Subsystem/If Action Subsystem15 ==
  Action Port : ActionPort  ActionType=else
  Constant : Constant  Value=21  OutDataTypeStr=uint8
  ThdRwRtStBkReclnEn_Clear : FunctionCaller  FunctionPrototype=ThdRwRtStBkReclnEn_Clear(data)  InputArgumentSpecifications=uint8(1)
  wires:
  Constant/1 -> ThdRwRtStBkReclnEn_Clear/1

== system Md58StEnCtrl/Md58StEnCtrl_Cal_sys/Subsystem/If Action Subsystem16 ==
  Action Port : ActionPort  ActionType=then
  Constant : Constant  Value=21  OutDataTypeStr=uint8
  ThdRwRtStBkReclnEn_Set : FunctionCaller  FunctionPrototype=ThdRwRtStBkReclnEn_Set(data)  InputArgumentSpecifications=uint8(1)
  wires:
  Constant/1 -> ThdRwRtStBkReclnEn_Set/1

== system Md58StEnCtrl/Md58StEnCtrl_Cal_sys/Subsystem/If Action Subsystem17 ==
  Action Port : ActionPort  ActionType=else
  Constant : Constant  Value=21  OutDataTypeStr=uint8
  ThdRwRtStFwdBkwdEn_Clear : FunctionCaller  FunctionPrototype=ThdRwRtStFwdBkwdEn_Clear(data)  InputArgumentSpecifications=uint8(1)
  wires:
  Constant/1 -> ThdRwRtStFwdBkwdEn_Clear/1

== system Md58StEnCtrl/Md58StEnCtrl_Cal_sys/Subsystem/If Action Subsystem18 ==
  Action Port : ActionPort  ActionType=then
  Constant : Constant  Value=21  OutDataTypeStr=uint8
  ThdRwRtStFwdBkwdEn_Set : FunctionCaller  FunctionPrototype=ThdRwRtStFwdBkwdEn_Set(data)  InputArgumentSpecifications=uint8(1)
  wires:
  Constant/1 -> ThdRwRtStFwdBkwdEn_Set/1

== system Md58StEnCtrl/Md58StEnCtrl_Cal_sys/Subsystem/If Action Subsystem19 ==
  Action Port : ActionPort  ActionType=else
  Constant : Constant  Value=21  OutDataTypeStr=uint8
  PassStFwdBkwdEn_Clear : FunctionCaller  FunctionPrototype=PassStFwdBkwdEn_Clear(data)  InputArgumentSpecifications=uint8(1)
  wires:
  Constant/1 -> PassStFwdBkwdEn_Clear/1

== system Md58StEnCtrl/Md58StEnCtrl_Cal_sys/Subsystem/If Action Subsystem2 ==
  Action Port : ActionPort  ActionType=then
  Constant : Constant  Value=21  OutDataTypeStr=uint8
  SecRwRtStFwdBkwdEn_Set : FunctionCaller  FunctionPrototype=SecRwRtStFwdBkwdEn_Set(data)  InputArgumentSpecifications=uint8(1)
  wires:
  Constant/1 -> SecRwRtStFwdBkwdEn_Set/1

== system Md58StEnCtrl/Md58StEnCtrl_Cal_sys/Subsystem/If Action Subsystem20 ==
  Action Port : ActionPort  ActionType=then
  Constant : Constant  Value=21  OutDataTypeStr=uint8
  PassStFwdBkwdEn_Set : FunctionCaller  FunctionPrototype=PassStFwdBkwdEn_Set(data)  InputArgumentSpecifications=uint8(1)
  wires:
  Constant/1 -> PassStFwdBkwdEn_Set/1

== system Md58StEnCtrl/Md58StEnCtrl_Cal_sys/Subsystem/If Action Subsystem21 ==
  Action Port : ActionPort  ActionType=else
  Constant : Constant  Value=21  OutDataTypeStr=uint8
  PassStBkReclnEn_Clear : FunctionCaller  FunctionPrototype=PassStBkReclnEn_Clear(data)  InputArgumentSpecifications=uint8(1)
  wires:
  Constant/1 -> PassStBkReclnEn_Clear/1

== system Md58StEnCtrl/Md58StEnCtrl_Cal_sys/Subsystem/If Action Subsystem22 ==
  Action Port : ActionPort  ActionType=then
  Constant : Constant  Value=21  OutDataTypeStr=uint8
  PassStBkReclnEn_Set : FunctionCaller  FunctionPrototype=PassStBkReclnEn_Set(data)  InputArgumentSpecifications=uint8(1)
  wires:
  Constant/1 -> PassStBkReclnEn_Set/1

== system Md58StEnCtrl/Md58StEnCtrl_Cal_sys/Subsystem/If Action Subsystem23 ==
  Action Port : ActionPort  ActionType=else
  Constant : Constant  Value=21  OutDataTypeStr=uint8
  PassStCshnFldEn_Clear : FunctionCaller  FunctionPrototype=PassStCshnFldEn_Clear(data)  InputArgumentSpecifications=uint8(1)
  wires:
  Constant/1 -> PassStCshnFldEn_Clear/1

== system Md58StEnCtrl/Md58StEnCtrl_Cal_sys/Subsystem/If Action Subsystem24 ==
  Action Port : ActionPort  ActionType=then
  Constant : Constant  Value=21  OutDataTypeStr=uint8
  PassStCshnFldEn_Set : FunctionCaller  FunctionPrototype=PassStCshnFldEn_Set(data)  InputArgumentSpecifications=uint8(1)
  wires:
  Constant/1 -> PassStCshnFldEn_Set/1

== system Md58StEnCtrl/Md58StEnCtrl_Cal_sys/Subsystem/If Action Subsystem3 ==
  note: Delete block
  note: Delete block
  Action Port : ActionPort  ActionType=else
  Constant : Constant  Value=21  OutDataTypeStr=uint8
  ThdRwLtStBkReclnEn_Clear : FunctionCaller  FunctionPrototype=ThdRwLtStBkReclnEn_Clear(data)  InputArgumentSpecifications=uint8(1)
  wires:
  Constant/1 -> ThdRwLtStBkReclnEn_Clear/1

== system Md58StEnCtrl/Md58StEnCtrl_Cal_sys/Subsystem/If Action Subsystem4 ==
  note: Delete block
  note: Delete block
  Action Port : ActionPort  ActionType=then
  Constant : Constant  Value=21  OutDataTypeStr=uint8
  ThdRwLtStBkReclnEn_Set : FunctionCaller  FunctionPrototype=ThdRwLtStBkReclnEn_Set(data)  InputArgumentSpecifications=uint8(1)
  wires:
  Constant/1 -> ThdRwLtStBkReclnEn_Set/1

== system Md58StEnCtrl/Md58StEnCtrl_Cal_sys/Subsystem/If Action Subsystem5 ==
  note: Delete block
  note: Delete block
  Action Port : ActionPort  ActionType=else
  Constant : Constant  Value=21  OutDataTypeStr=uint8
  ThdRwLtStFwdBkwdEn_Clear : FunctionCaller  FunctionPrototype=ThdRwLtStFwdBkwdEn_Clear(data)  InputArgumentSpecifications=uint8(1)
  wires:
  Constant/1 -> ThdRwLtStFwdBkwdEn_Clear/1
